simulink model "first_block"  (R2022a)
settings: Solver=VariableStepAuto  StartTime=0.0  StopTime=10.0  RelTol=1e-3
libraries: simulink x3
settings Model: Creator=User  LastModifiedBy=User

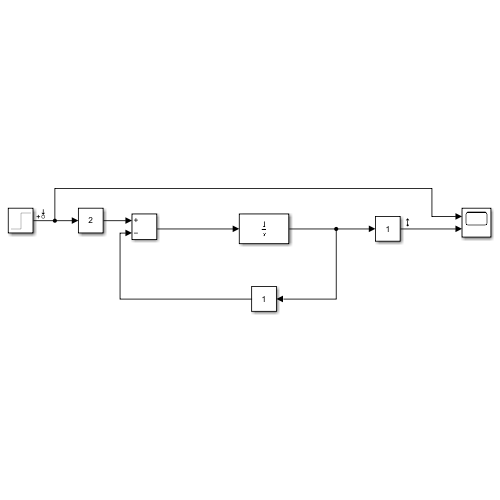
[thumbnail: Simulink's stored preview of the top-level diagram]
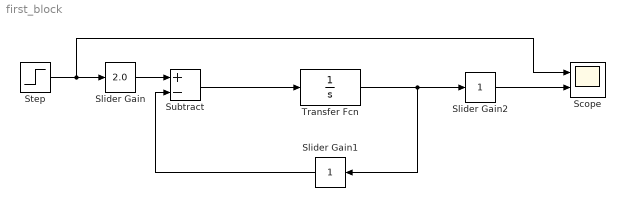
== system first_block ==
  Scope : Scope  NumInputPorts=2
  Slider Gain : simulink/Math Operations/Slider Gain  gain=2.0  low=0  high=2
  Slider Gain1 : simulink/Math Operations/Slider Gain  gain=1  low=-1  high=2
  Slider Gain2 : simulink/Math Operations/Slider Gain  gain=1  low=0  high=2
  Step : Step  SampleTime=0
  Subtract : Sum  Inputs=+-
  Transfer Fcn : TransferFcn  Numerator=1  Denominator=[1 0]  ContinuousStateAttributes="''K_ии/s\""
  wires:
  Step/1 -> Scope/1, Slider Gain/1
  Slider Gain/1 -> Subtract/1
  Subtract/1 -> Transfer Fcn/1
  Transfer Fcn/1 -> Slider Gain2/1, Slider Gain1/1
  Slider Gain1/1 -> Subtract/2
  Slider Gain2/1 -> Scope/2
